simulink model "Lab1_parameter_estimation_student"  (R2025a)
settings: Solver=FixedStepAuto  StartTime=0.0  StopTime=inf  FixedStep=0.001  RelTol=1e-3
values from neighbouring files (symbols this model uses):
  Chirmp_Time = 20.5    [Cross_Validation.m]
  Mode = 5    [Cross_Validation.m]
  motor_B = 8.54E-06    (= 8.54e-06)    [Lab1_motor_params_student.m]    (also in Lab_1_parameter_generate.m = 3.9e-06)
  motor_Eff = 0.92042    [Lab1_motor_params_student.m]    (also in Lab_1_parameter_generate.m = 0.8279549717)
  motor_J = 1/6382.937317    (= 0.00015666768297)    [Lab1_motor_params_student.m]    (also in Lab_1_parameter_generate.m = 0.05438258655)
  motor_Ke = 0.05438258655    [Lab1_motor_params_student.m]    (also in Lab_1_parameter_generate.m = 6382.937317)
  motor_L = 0.02587    [Lab1_motor_params_student.m]    (also in Lab_1_parameter_generate.m = 0.002587)
  motor_R = 3.341    [Lab1_motor_params_student.m]    (also in Lab_1_parameter_generate.m)
  Ramp_Slope = 0.05    [Cross_Validation.m]
  Sine_Freq = pi/4    (= 0.785398163397)    [Cross_Validation.m]
  Stair_Wait = 2    [Cross_Validation.m]
  Step_Value = 1    [Cross_Validation.m]
libraries: simulink x2
settings Model: Creator=tanawatp  LastModifiedBy=ACER
settings DataIOCC: OutputOption=AdditionalOutputTimes  OutputTimes=SDO_OutputTimes  ReturnWorkspaceOutputsName=SDOSimTest_Log
settings RTWCC: GPUComputeCapability=3.5

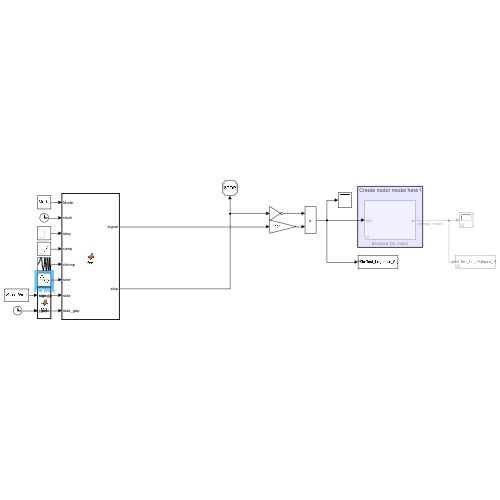
[thumbnail: Simulink's stored preview of the top-level diagram]
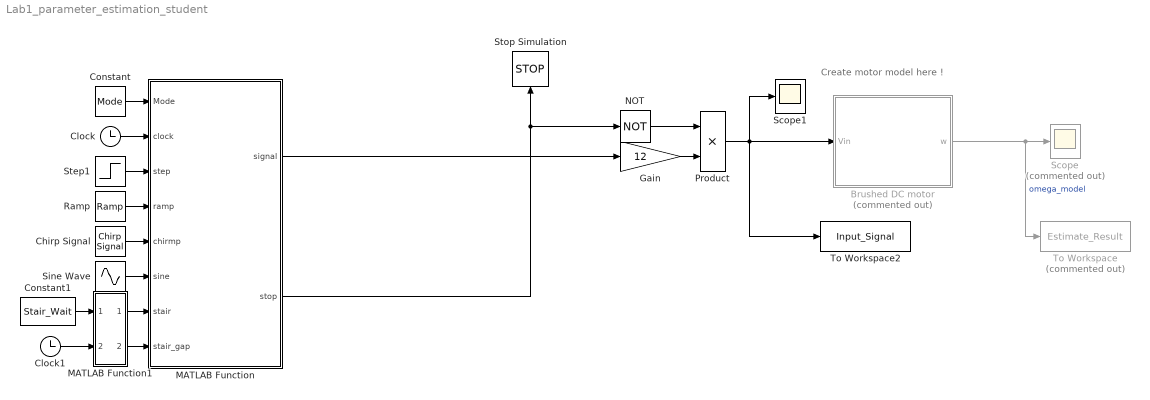
== system Lab1_parameter_estimation_student ==
  note: Create motor model here !
  Brushed DC motor : Subsystem  Commented=on
  Chirp Signal : simulink/Sources/Chirp Signal  f1=0  T=Chirmp_Time  f2=Chirmp_Freq
  Clock : Clock
  Clock1 : Clock
  Constant : Constant  Value=Mode
  Constant1 : Constant  Value=Stair_Wait
  Gain : Gain  Gain=12
  MATLAB Function : MATLAB Function  TreatAsAtomicUnit=on
  MATLAB Function1 : MATLAB Function  TreatAsAtomicUnit=on
  NOT : Logic  Operator=NOT  IconShape=distinctive  AllPortsSameDT=off  OutDataTypeStr=boolean
  Product : Product
  Ramp : simulink/Sources/Ramp  slope=Ramp_Slope  start=0.5  InitialOutput=-1
  Scope : Scope  Commented=on
      settings: ActiveDisplayYMinimum=-0.04476959904659604  ActiveDisplayYMaximum=0.061841059230423143
  Scope1 : Scope
      settings: ActiveDisplayYMinimum=-0.04476959904659604  ActiveDisplayYMaximum=0.061841059230423143
  Sine Wave : Sin  Frequency=Sine_Freq  SampleTime=0
  Step1 : Step  Time=0.5  After=Step_Value  SampleTime=0
  Stop Simulation : Stop
  To Workspace : ToWorkspace  Commented=on  VariableName=Estimate_Result  SaveFormat=Structure With Time  SampleTime=-1
  To Workspace2 : ToWorkspace  VariableName=Input_Signal  SaveFormat=Structure With Time  SampleTime=-1
  wires:
  Brushed DC motor/1(w) -> To Workspace/1, Scope/1  "omega_model"
  Product/1 -> Scope1/1, To Workspace2/1, Brushed DC motor/1(Vin)
  Clock1/1 -> MATLAB Function1/2(clock)
  MATLAB Function1/1(signal) -> MATLAB Function/7(stair)
  MATLAB Function/2(stop) -> NOT/1, Stop Simulation/1
  MATLAB Function1/2(stair_gaps) -> MATLAB Function/8(stair_gap)
  Constant1/1 -> MATLAB Function1/1(stair_gap)
  Chirp Signal/1 -> MATLAB Function/5(chirmp)
  MATLAB Function/1(signal) -> Gain/1
  Constant/1 -> MATLAB Function/1(Mode)
  Sine Wave/1 -> MATLAB Function/6(sine)
  Ramp/1 -> MATLAB Function/4(ramp)
  Clock/1 -> MATLAB Function/2(clock)
  Step1/1 -> MATLAB Function/3(step)
  Gain/1 -> Product/2
  NOT/1 -> Product/1

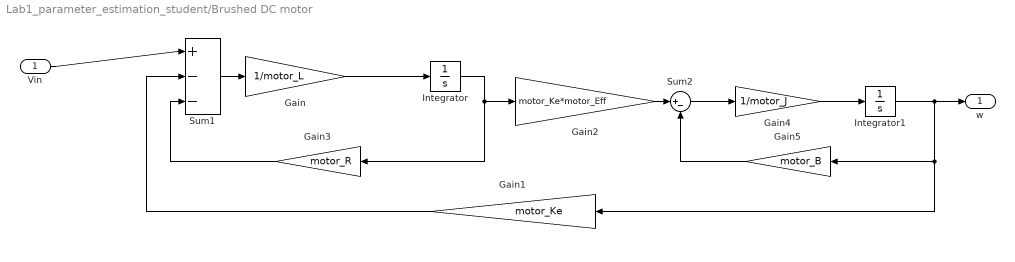
== system Lab1_parameter_estimation_student/Brushed DC motor ==
  Vin : Inport
  Gain : Gain  Gain=1/motor_L
  Gain1 : Gain  Gain=motor_Ke
  Gain2 : Gain  Gain=motor_Ke*motor_Eff
  Gain3 : Gain  Gain=motor_R
  Gain4 : Gain  Gain=1/motor_J
  Gain5 : Gain  Gain=motor_B
  Integrator : Integrator
  Integrator1 : Integrator
  Sum1 : Sum  Inputs=|+--
  Sum2 : Sum  Inputs=|+-
  w : Outport
  wires:
  Vin/1 -> Sum1/1
  Sum1/1 -> Gain/1
  Integrator/1 -> Gain3/1, Gain2/1
  Gain3/1 -> Sum1/3
  Sum2/1 -> Gain4/1
  Gain2/1 -> Sum2/1
  Integrator1/1 -> Gain1/1, Gain5/1, w/1
  Gain5/1 -> Sum2/2
  Gain1/1 -> Sum1/2
  Gain4/1 -> Integrator1/1
  Gain/1 -> Integrator/1

== matlab function Lab1_parameter_estimation_student/MATLAB Function1 ==
  data: signal output; stair_gaps output; stair_gap input; clock input
function [signal,stair_gaps]= fcn(stair_gap,clock)
time_offset = 0.5;
All_signal = 0.1:0.1:1;
clock_usage = clock - time_offset;
if clock_usage < 0
    clock_usage = 0;
end
phase = fix(clock_usage/stair_gap/2);
stair_gaps = stair_gap;
if clock < 0.5
    signal = 0;
    return;
end

if phase <= 9
    buffer = clock_usage - 2*stair_gap*phase;
    if buffer < stair_gap
        signal = All_signal(phase+1);
    else
        signal = 0;
    end
else
    signal = 0;
end

    end

== matlab function Lab1_parameter_estimation_student/MATLAB Function ==
  data: Mode input; signal output; clock input; step input; ramp input; chirmp input; sine input; stair input; stop output; stair_gap input
function [signal, stop] = fcn(Mode, clock, step, ramp, chirmp, sine, stair, stair_gap)

% Default outputs
signal = 0;
stop   = 0;

% Initial 0.5 sec zero output
if clock < 0.5
    return;
end

switch Mode

    case 1   % STEP
        signal = step;
        if clock >= 10.5
            stop = 1;
        end

    case 2   % RAMP
        signal = ramp;
        if signal >= 1
            stop = 1;
        end

    case 3   % CHIRP
        signal = chirmp;
        if clock >= 10.5
            stop = 1;
        end

    case 4   % SINE
        signal = sine;
        if clock >= 10.5
            stop = 1;
        end

  case 5   % STAIR
        signal = stair;

        % 10 amplitudes × (ON + OFF) × stair_gap + 0.5 sec initial
        total_time = 0.6 + 20 * stair_gap;

        if clock >= total_time
            stop = 1;
        end

    otherwise
        signal = 0;
        stop   = 0;
end

end
